simulink library "pack_5p48s8p_1g10g1_Iso_library"  (R2026a)
settings: Solver=VariableStepAuto
undefined symbols (not defined in the file or in its folder): batt_5p48s_1g10g1_thr, battery_builder_rtmsupport, gcbh, ModuleAssembly1, ModuleType1, plate_5p48s_1g10g1_thr, targets_5p48s8p_1g10g1_thr
libraries: $bdroot x8, pack_5p48s8p_1g10g1_Iso_lib x4
Description:
  | Copyright 2023-2026 The MathWorks, Inc.
settings Model: Creator=smiller  LastModifiedBy=smiller

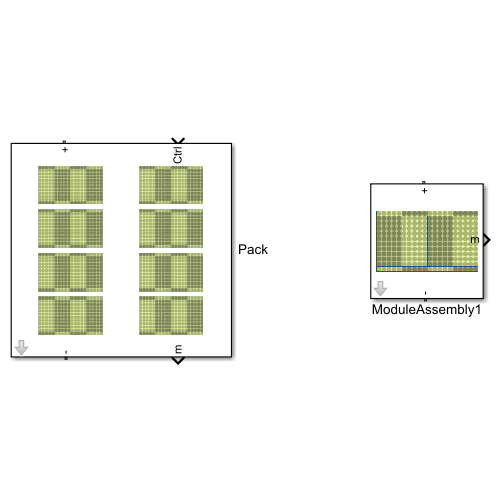
[thumbnail: Simulink's stored preview of the top-level diagram]
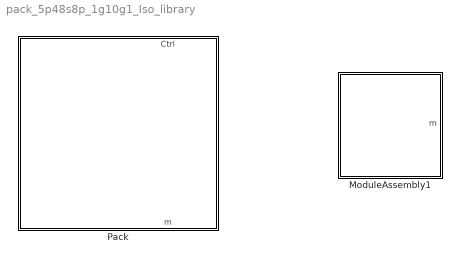
== system pack_5p48s8p_1g10g1_Iso_library ==
  ModuleAssembly1 : Subsystem  LoadFcn=battery_builder_rtmsupport('loadfcn',gcbh);  mask{Cell=ModuleType1, Targets=ModuleAssembly1, BatteryObj=batt_5p48s_1g10g1_thr}
      mask prompts: Cell "Cell Parameters"; Targets "Cell Targets"; BatteryObj "Battery Object"
      settings: PreCopyFcn=battery_builder_rtmsupport('precopyfcn',gcbh);  PreDeleteFcn=battery_builder_rtmsupport('predeletefcn',gcbh);  PortSchema="{\"entries\":[{\"content\":{\"sides\":[{\"content\":{\"connectorIds\":[\"LConn1\"]},\"type\":\"ConnectorPlacement.EquallySpacedRectSide\",\"uuid\":\"bc91a472-35c0-4041-89a6-b649b08794f0\"},{\"content\":{\"connectorIds\":[\"RConn1\"],\"side\":\"RIGHT\"},\"type\":\"ConnectorPlacement.EquallySpacedRectSide\",\"uuid\":\"4a390b53-12a2-4d2f-9537-abc76db307f8\"},{\"content\":{\"connectorIds\":[],\"side\":\"TOP\"},\"type\":\"ConnectorPlacement.EquallySpacedRectSide\",\"uuid\":\"1a7ed896-4ada-4d88-995c-c24bd39ee86b\"},{\"content\":{\"connectorIds\":[\"Out1\"],\"side\":\"BOTTOM\"},\"type\":\"ConnectorPlacement.EquallySpacedRectSide\",\"uuid\":\"e36c911b-adc9-44cf-bfab-32777b2ec35c\"}]},\"type\":\"ConnectorPlacement.EquallySpacedConnector\",\"uuid\":\"4e67d65b-f12d-4d00-91b0-7eadb0a42625\"}],\"packageUris\":[\"http://schema.mathworks.com/mf0/Connector/R2020b\"],\"version\":\"1.0\"}"
      mask Display: image('module_5p48s_1g10g1_IMAGE.png')
  Pack : Subsystem  LoadFcn=battery_builder_rtmsupport('loadfcn',gcbh);  mask{cell_param=ModuleType1, targets=targets_5p48s8p_1g10g1_thr, plate=plate_5p48s_1g10g1_thr, batt_obj=batt_5p48s_1g10g1_thr}
      mask prompts: cell_param "Cell Parameters"; targets "Cell Targets"; plate "Plate Parameters"; batt_obj "Battery Object"
      settings: PreCopyFcn=battery_builder_rtmsupport('precopyfcn',gcbh);  PreDeleteFcn=battery_builder_rtmsupport('predeletefcn',gcbh);
      mask Display: image('pack_5p48s8p_1g10g1_IMAGE.png')

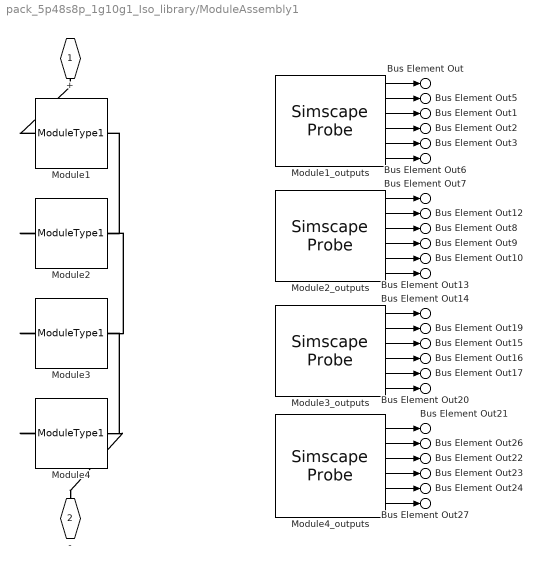
== system pack_5p48s8p_1g10g1_Iso_library/ModuleAssembly1 ==
  Module1 : pack_5p48s8p_1g10g1_Iso_lib/Modules/ModuleType1  BatteryCapacityCell=ModuleType1.BatteryCapacityCell A*hr  ExtrapolationMethodCell=simscape.enum.extrapolation.nearest  SOCBreakpointsCell=ModuleType1.SOCBreakpointsCell  TemperatureBreakpointsCell=ModuleType1.TemperatureBreakpointsCell K  OpenCircuitVoltageThermalCell=ModuleType1.OpenCircuitVoltageThermalCell V  VoltageRangeCell=ModuleType1.VoltageRangeCell V  ResistanceSOCBreakpointsCell=ModuleType1.ResistanceSOCBreakpointsCell  ResistanceTemperatureBreakpointsCell=ModuleType1.ResistanceTemperatureBreakpointsCell K  R0ThermalCell=ModuleType1.R0ThermalCell Ohm  SimulationTemperatureCell=ModuleType1.SimulationTemperatureCell K  socCell_specify=off  socCell_priority=High  socCell=repmat(1, 3, 1)  socCell_nominal_specify=off  socCell_nominal_value=1  socCell_nominal_unit=1  batteryVoltage_specify=off  batteryVoltage_priority=None  batteryVoltage=repmat(0, 3, 1) V  batteryVoltage_nominal_specify=off  batteryVoltage_nominal_value=1  batteryVoltage_nominal_unit=V  batteryCurrent_specify=off  batteryCurrent_priority=None  batteryCurrent=repmat(0, 3, 1) A  batteryCurrent_nominal_specify=off  batteryCurrent_nominal_value=1  batteryCurrent_nominal_unit=A  numCycles_specify=off  numCycles_priority=High  numCycles=repmat(0, 3, 1)  numCycles_nominal_specify=off  numCycles_nominal_value=1  numCycles_nominal_unit=1  vParallelAssembly_specify=on  vParallelAssembly_priority=None  vParallelAssembly=Targets.Module1.vParallelAssembly V  vParallelAssembly_nominal_specify=off  vParallelAssembly_nominal_value=1  vParallelAssembly_nominal_unit=V  socParallelAssembly_specify=on  socParallelAssembly_priority=None  socParallelAssembly=Targets.Module1.socParallelAssembly  socParallelAssembly_nominal_specify=off  socParallelAssembly_nominal_value=1  socParallelAssembly_nominal_unit=1
  Module1_outputs : SimscapeProbe  BoundBlock=1177  Variables="{\"batteryCurrent\":{\"Probing\":\"ON\"},\"batteryVoltage\":{\"Probing\":\"ON\"},\"iCell\":{\"Probing\":\"OFF\"},\"numCycles\":{\"Probing\":\"ON\"},\"numCyclesCell\":{\"Probing\":\"OFF\"},\"socCell\":{\"Probing\":\"ON\"},\"socParallelAssembly\":{\"Probing\":\"ON\"},\"vCell\":{\"Probing\":\"OFF\"},\"vParallelAssembly\":{\"Probing\":\"ON\"}}"
  Module2 : pack_5p48s8p_1g10g1_Iso_lib/Modules/ModuleType1  BatteryCapacityCell=ModuleType1.BatteryCapacityCell A*hr  ExtrapolationMethodCell=simscape.enum.extrapolation.nearest  SOCBreakpointsCell=ModuleType1.SOCBreakpointsCell  TemperatureBreakpointsCell=ModuleType1.TemperatureBreakpointsCell K  OpenCircuitVoltageThermalCell=ModuleType1.OpenCircuitVoltageThermalCell V  VoltageRangeCell=ModuleType1.VoltageRangeCell V  ResistanceSOCBreakpointsCell=ModuleType1.ResistanceSOCBreakpointsCell  ResistanceTemperatureBreakpointsCell=ModuleType1.ResistanceTemperatureBreakpointsCell K  R0ThermalCell=ModuleType1.R0ThermalCell Ohm  SimulationTemperatureCell=ModuleType1.SimulationTemperatureCell K  socCell_specify=off  socCell_priority=High  socCell=repmat(1, 3, 1)  socCell_nominal_specify=off  socCell_nominal_value=1  socCell_nominal_unit=1  batteryVoltage_specify=off  batteryVoltage_priority=None  batteryVoltage=repmat(0, 3, 1) V  batteryVoltage_nominal_specify=off  batteryVoltage_nominal_value=1  batteryVoltage_nominal_unit=V  batteryCurrent_specify=off  batteryCurrent_priority=None  batteryCurrent=repmat(0, 3, 1) A  batteryCurrent_nominal_specify=off  batteryCurrent_nominal_value=1  batteryCurrent_nominal_unit=A  numCycles_specify=off  numCycles_priority=High  numCycles=repmat(0, 3, 1)  numCycles_nominal_specify=off  numCycles_nominal_value=1  numCycles_nominal_unit=1  vParallelAssembly_specify=on  vParallelAssembly_priority=None  vParallelAssembly=Targets.Module2.vParallelAssembly V  vParallelAssembly_nominal_specify=off  vParallelAssembly_nominal_value=1  vParallelAssembly_nominal_unit=V  socParallelAssembly_specify=on  socParallelAssembly_priority=None  socParallelAssembly=Targets.Module2.socParallelAssembly  socParallelAssembly_nominal_specify=off  socParallelAssembly_nominal_value=1  socParallelAssembly_nominal_unit=1
  Module2_outputs : SimscapeProbe  BoundBlock=1178  Variables="{\"batteryCurrent\":{\"Probing\":\"ON\"},\"batteryVoltage\":{\"Probing\":\"ON\"},\"iCell\":{\"Probing\":\"OFF\"},\"numCycles\":{\"Probing\":\"ON\"},\"numCyclesCell\":{\"Probing\":\"OFF\"},\"socCell\":{\"Probing\":\"ON\"},\"socParallelAssembly\":{\"Probing\":\"ON\"},\"vCell\":{\"Probing\":\"OFF\"},\"vParallelAssembly\":{\"Probing\":\"ON\"}}"
  Module3 : pack_5p48s8p_1g10g1_Iso_lib/Modules/ModuleType1  BatteryCapacityCell=ModuleType1.BatteryCapacityCell A*hr  ExtrapolationMethodCell=simscape.enum.extrapolation.nearest  SOCBreakpointsCell=ModuleType1.SOCBreakpointsCell  TemperatureBreakpointsCell=ModuleType1.TemperatureBreakpointsCell K  OpenCircuitVoltageThermalCell=ModuleType1.OpenCircuitVoltageThermalCell V  VoltageRangeCell=ModuleType1.VoltageRangeCell V  ResistanceSOCBreakpointsCell=ModuleType1.ResistanceSOCBreakpointsCell  ResistanceTemperatureBreakpointsCell=ModuleType1.ResistanceTemperatureBreakpointsCell K  R0ThermalCell=ModuleType1.R0ThermalCell Ohm  SimulationTemperatureCell=ModuleType1.SimulationTemperatureCell K  socCell_specify=off  socCell_priority=High  socCell=repmat(1, 3, 1)  socCell_nominal_specify=off  socCell_nominal_value=1  socCell_nominal_unit=1  batteryVoltage_specify=off  batteryVoltage_priority=None  batteryVoltage=repmat(0, 3, 1) V  batteryVoltage_nominal_specify=off  batteryVoltage_nominal_value=1  batteryVoltage_nominal_unit=V  batteryCurrent_specify=off  batteryCurrent_priority=None  batteryCurrent=repmat(0, 3, 1) A  batteryCurrent_nominal_specify=off  batteryCurrent_nominal_value=1  batteryCurrent_nominal_unit=A  numCycles_specify=off  numCycles_priority=High  numCycles=repmat(0, 3, 1)  numCycles_nominal_specify=off  numCycles_nominal_value=1  numCycles_nominal_unit=1  vParallelAssembly_specify=on  vParallelAssembly_priority=None  vParallelAssembly=Targets.Module3.vParallelAssembly V  vParallelAssembly_nominal_specify=off  vParallelAssembly_nominal_value=1  vParallelAssembly_nominal_unit=V  socParallelAssembly_specify=on  socParallelAssembly_priority=None  socParallelAssembly=Targets.Module3.socParallelAssembly  socParallelAssembly_nominal_specify=off  socParallelAssembly_nominal_value=1  socParallelAssembly_nominal_unit=1
  Module3_outputs : SimscapeProbe  BoundBlock=1179  Variables="{\"batteryCurrent\":{\"Probing\":\"ON\"},\"batteryVoltage\":{\"Probing\":\"ON\"},\"iCell\":{\"Probing\":\"OFF\"},\"numCycles\":{\"Probing\":\"ON\"},\"numCyclesCell\":{\"Probing\":\"OFF\"},\"socCell\":{\"Probing\":\"ON\"},\"socParallelAssembly\":{\"Probing\":\"ON\"},\"vCell\":{\"Probing\":\"OFF\"},\"vParallelAssembly\":{\"Probing\":\"ON\"}}"
  Module4 : pack_5p48s8p_1g10g1_Iso_lib/Modules/ModuleType1  BatteryCapacityCell=ModuleType1.BatteryCapacityCell A*hr  ExtrapolationMethodCell=simscape.enum.extrapolation.nearest  SOCBreakpointsCell=ModuleType1.SOCBreakpointsCell  TemperatureBreakpointsCell=ModuleType1.TemperatureBreakpointsCell K  OpenCircuitVoltageThermalCell=ModuleType1.OpenCircuitVoltageThermalCell V  VoltageRangeCell=ModuleType1.VoltageRangeCell V  ResistanceSOCBreakpointsCell=ModuleType1.ResistanceSOCBreakpointsCell  ResistanceTemperatureBreakpointsCell=ModuleType1.ResistanceTemperatureBreakpointsCell K  R0ThermalCell=ModuleType1.R0ThermalCell Ohm  SimulationTemperatureCell=ModuleType1.SimulationTemperatureCell K  socCell_specify=off  socCell_priority=High  socCell=repmat(1, 3, 1)  socCell_nominal_specify=off  socCell_nominal_value=1  socCell_nominal_unit=1  batteryVoltage_specify=off  batteryVoltage_priority=None  batteryVoltage=repmat(0, 3, 1) V  batteryVoltage_nominal_specify=off  batteryVoltage_nominal_value=1  batteryVoltage_nominal_unit=V  batteryCurrent_specify=off  batteryCurrent_priority=None  batteryCurrent=repmat(0, 3, 1) A  batteryCurrent_nominal_specify=off  batteryCurrent_nominal_value=1  batteryCurrent_nominal_unit=A  numCycles_specify=off  numCycles_priority=High  numCycles=repmat(0, 3, 1)  numCycles_nominal_specify=off  numCycles_nominal_value=1  numCycles_nominal_unit=1  vParallelAssembly_specify=on  vParallelAssembly_priority=None  vParallelAssembly=Targets.Module3.vParallelAssembly V  vParallelAssembly_nominal_specify=off  vParallelAssembly_nominal_value=1  vParallelAssembly_nominal_unit=V  socParallelAssembly_specify=on  socParallelAssembly_priority=None  socParallelAssembly=Targets.Module3.socParallelAssembly  socParallelAssembly_nominal_specify=off  socParallelAssembly_nominal_value=1  socParallelAssembly_nominal_unit=1
  Module4_outputs : SimscapeProbe  BoundBlock=1180  Variables="{\"batteryCurrent\":{\"Probing\":\"ON\"},\"batteryVoltage\":{\"Probing\":\"ON\"},\"iCell\":{\"Probing\":\"OFF\"},\"numCycles\":{\"Probing\":\"ON\"},\"numCyclesCell\":{\"Probing\":\"OFF\"},\"socCell\":{\"Probing\":\"ON\"},\"socParallelAssembly\":{\"Probing\":\"ON\"},\"vCell\":{\"Probing\":\"OFF\"},\"vParallelAssembly\":{\"Probing\":\"ON\"}}"
  + : PMIOPort  Side=Left
  - : PMIOPort  Port=2  Side=Right
  Bus Element Out : Outport  PortName=m  Element=i.M1
  Bus Element Out7 : Outport  PortName=m  Element=i.M2
  Bus Element Out14 : Outport  PortName=m  Element=i.M3
  Bus Element Out21 : Outport  PortName=m  Element=i.M4
  Bus Element Out1 : Outport  PortName=m  Element=cyc.M1
  Bus Element Out8 : Outport  PortName=m  Element=cyc.M2
  Bus Element Out15 : Outport  PortName=m  Element=cyc.M3
  Bus Element Out22 : Outport  PortName=m  Element=cyc.M4
  Bus Element Out2 : Outport  PortName=m  Element=socC.M1
  Bus Element Out9 : Outport  PortName=m  Element=socC.M2
  Bus Element Out16 : Outport  PortName=m  Element=socC.M3
  Bus Element Out23 : Outport  PortName=m  Element=socC.M4
  Bus Element Out3 : Outport  PortName=m  Element=socP.M1
  Bus Element Out10 : Outport  PortName=m  Element=socP.M2
  Bus Element Out17 : Outport  PortName=m  Element=socP.M3
  Bus Element Out24 : Outport  PortName=m  Element=socP.M4
  Bus Element Out5 : Outport  PortName=m  Element=vC.M1
  Bus Element Out12 : Outport  PortName=m  Element=vC.M2
  Bus Element Out19 : Outport  PortName=m  Element=vC.M3
  Bus Element Out26 : Outport  PortName=m  Element=vC.M4
  Bus Element Out6 : Outport  PortName=m  Element=vP.M1
  Bus Element Out13 : Outport  PortName=m  Element=vP.M2
  Bus Element Out20 : Outport  PortName=m  Element=vP.M3
  Bus Element Out27 : Outport  PortName=m  Element=vP.M4
  wires:
  Module1_outputs/1 -> Bus Element Out/1
  Module1_outputs/2 -> Bus Element Out5/1
  Module1_outputs/3 -> Bus Element Out1/1
  Module1_outputs/4 -> Bus Element Out2/1
  Module1_outputs/5 -> Bus Element Out3/1
  Module1_outputs/6 -> Bus Element Out6/1
  Module2_outputs/1 -> Bus Element Out7/1
  Module2_outputs/2 -> Bus Element Out12/1
  Module2_outputs/3 -> Bus Element Out8/1
  Module2_outputs/4 -> Bus Element Out9/1
  Module2_outputs/5 -> Bus Element Out10/1
  Module2_outputs/6 -> Bus Element Out13/1
  Module3_outputs/1 -> Bus Element Out14/1
  Module3_outputs/2 -> Bus Element Out19/1
  Module3_outputs/3 -> Bus Element Out15/1
  Module3_outputs/4 -> Bus Element Out16/1
  Module3_outputs/5 -> Bus Element Out17/1
  Module3_outputs/6 -> Bus Element Out20/1
  Module4_outputs/1 -> Bus Element Out21/1
  Module4_outputs/2 -> Bus Element Out26/1
  Module4_outputs/3 -> Bus Element Out22/1
  Module4_outputs/4 -> Bus Element Out23/1
  Module4_outputs/5 -> Bus Element Out24/1
  Module4_outputs/6 -> Bus Element Out27/1
  connections:
  Module1/LConn1 -- +/RConn1
  Module4/RConn1 -- -/RConn1
  Module2/LConn1 -- Module1/RConn1
  Module3/LConn1 -- Module2/RConn1
  Module4/LConn1 -- Module3/RConn1

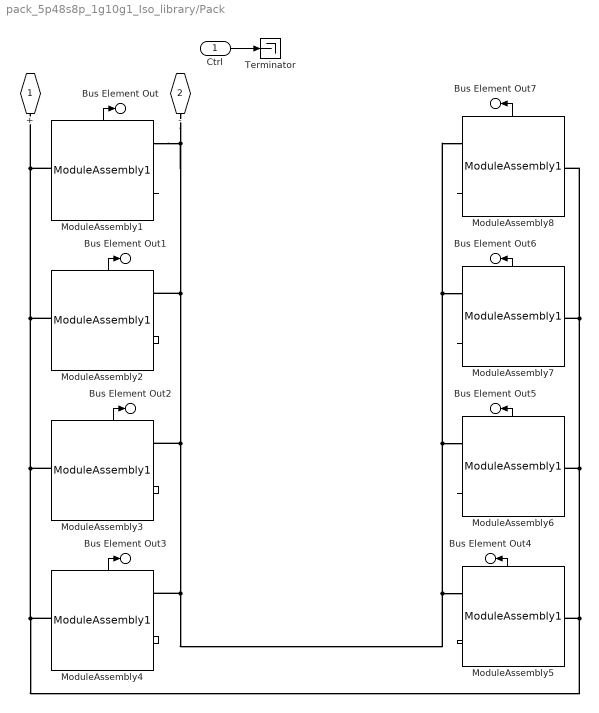
== system pack_5p48s8p_1g10g1_Iso_library/Pack ==
  Ctrl : Inport
  ModuleAssembly1 : $bdroot/ModuleAssembly1  Cell=cell_param  Targets=targets.ModuleAssembly1  BatteryObj=batt_obj
  ModuleAssembly2 : $bdroot/ModuleAssembly1  Cell=cell_param  Targets=targets.ModuleAssembly2  BatteryObj=batt_obj
  ModuleAssembly3 : $bdroot/ModuleAssembly1  Cell=cell_param  Targets=targets.ModuleAssembly3  BatteryObj=batt_obj
  ModuleAssembly4 : $bdroot/ModuleAssembly1  Cell=cell_param  Targets=targets.ModuleAssembly4  BatteryObj=batt_obj
  ModuleAssembly5 : $bdroot/ModuleAssembly1  Cell=cell_param  Targets=targets.ModuleAssembly5  BatteryObj=batt_obj
  ModuleAssembly6 : $bdroot/ModuleAssembly1  Cell=cell_param  Targets=targets.ModuleAssembly6  BatteryObj=batt_obj
  ModuleAssembly7 : $bdroot/ModuleAssembly1  Cell=cell_param  Targets=targets.ModuleAssembly7  BatteryObj=batt_obj
  ModuleAssembly8 : $bdroot/ModuleAssembly1  Cell=cell_param  Targets=targets.ModuleAssembly8  BatteryObj=batt_obj
  Terminator : Terminator
  + : PMIOPort  Side=Left
  - : PMIOPort  Port=2  Side=Right
  Bus Element Out : Outport  PortName=m  Element=A1
  Bus Element Out1 : Outport  PortName=m  Element=A2
  Bus Element Out2 : Outport  PortName=m  Element=A3
  Bus Element Out3 : Outport  PortName=m  Element=A4
  Bus Element Out4 : Outport  PortName=m  Element=A5
  Bus Element Out5 : Outport  PortName=m  Element=A6
  Bus Element Out6 : Outport  PortName=m  Element=A7
  Bus Element Out7 : Outport  PortName=m  Element=A8
  wires:
  ModuleAssembly1/1 -> Bus Element Out/1
  ModuleAssembly2/1 -> Bus Element Out1/1
  ModuleAssembly3/1 -> Bus Element Out2/1
  ModuleAssembly4/1 -> Bus Element Out3/1
  ModuleAssembly5/1 -> Bus Element Out4/1
  ModuleAssembly6/1 -> Bus Element Out5/1
  ModuleAssembly7/1 -> Bus Element Out6/1
  ModuleAssembly8/1 -> Bus Element Out7/1
  Ctrl/1 -> Terminator/1
  connections:
  ModuleAssembly1/RConn1 -- ModuleAssembly8/RConn1 -- ModuleAssembly7/RConn1 -- ModuleAssembly6/RConn1 -- ModuleAssembly5/RConn1 -- ModuleAssembly4/RConn1 -- ModuleAssembly3/RConn1 -- ModuleAssembly2/RConn1 -- -/RConn1
  ModuleAssembly1/LConn1 -- ModuleAssembly6/LConn1 -- ModuleAssembly8/LConn1 -- ModuleAssembly7/LConn1 -- ModuleAssembly5/LConn1 -- ModuleAssembly4/LConn1 -- ModuleAssembly3/LConn1 -- ModuleAssembly2/LConn1 -- +/RConn1
